simulink model "energy_recovery_testbench_r2024a"  (R2024a)
settings: Solver=daessc  StartTime=0  StopTime=0.4  MaxStep=1e-6  RelTol=1e-4
model workspace (MAT data in the model file):
  Fout_Hz = 50
  LoadEnable = 0
  RegenCurrentRef_RMS_A = 0.5
  RegenEnable = 1
  Rphase = 9.23760430703
libraries: fl_lib x38, nesl_utility x28
settings Model: Creator=chidan  LastModifiedBy=chidan

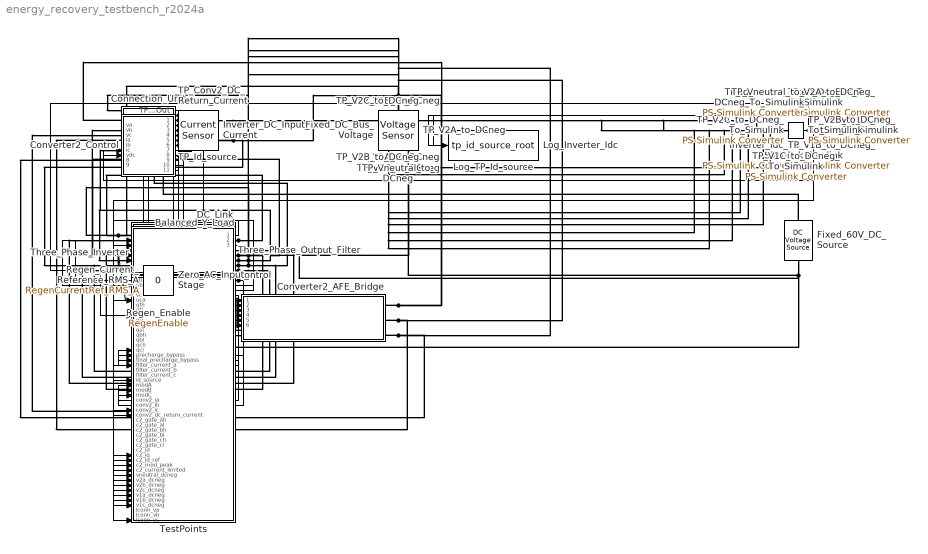
== system energy_recovery_testbench_r2024a ==
  Balanced_Y_Load : Subsystem
  Connection_Unit : Subsystem
  Control : Subsystem  ReferencedSubsystem=converter1_control_r2024a
  Converter2_AFE_Bridge : Subsystem  ReferencedSubsystem=converter1_inverter_r2024a
  Converter2_Control : Subsystem
  DC_Link : Subsystem
  Fixed_60V_DC_Source : fl_lib/Electrical/Electrical Sources/DC Voltage Source  v0=60 V
  Fixed_DC_Bus_To_Simulink : nesl_utility/PS-Simulink Converter  PhysicalDomain=network_engine_domain  SubClassName=ps_output  LeftPortType=input  RightPortType=output  PseudoPeriodic=off  Frequencies=[]  VectorFormat=inherit  Unit=V  AffineConversion=off
  Fixed_DC_Bus_Voltage : fl_lib/Electrical/Electrical Sensors/Voltage Sensor
  Inverter_DC_Input_Current : fl_lib/Electrical/Electrical Sensors/Current Sensor
  Inverter_Idc_To_Simulink : nesl_utility/PS-Simulink Converter  PhysicalDomain=network_engine_domain  SubClassName=ps_output  LeftPortType=input  RightPortType=output  PseudoPeriodic=off  Frequencies=[]  VectorFormat=inherit  Unit=A  AffineConversion=off
  Log_Inverter_Idc : ToWorkspace  VariableName=acac_idc_inverter  SaveFormat=Timeseries  SampleTime=-1
  Log_TP_Id_source : ToWorkspace  VariableName=tp_id_source_root  SaveFormat=Timeseries  SampleTime=-1
  Regen_Current_Reference_RMS_A : Constant  Value=RegenCurrentRef_RMS_A
  Regen_Enable : Constant  Value=RegenEnable
  TP_Conv2_DC_Return_Current : fl_lib/Electrical/Electrical Sensors/Current Sensor
  TP_Conv2_DC_Return_To_Simulink : nesl_utility/PS-Simulink Converter  PhysicalDomain=network_engine_domain  SubClassName=ps_output  LeftPortType=input  RightPortType=output  PseudoPeriodic=off  Frequencies=[]  VectorFormat=inherit  Unit=inherit  AffineConversion=off
  TP_Id_source : fl_lib/Electrical/Electrical Sensors/Current Sensor
  TP_Id_source_To_Simulink : nesl_utility/PS-Simulink Converter  PhysicalDomain=network_engine_domain  SubClassName=ps_output  LeftPortType=input  RightPortType=output  PseudoPeriodic=off  Frequencies=[]  VectorFormat=inherit  Unit=inherit  AffineConversion=off
  TP_V1A_to_DCneg : fl_lib/Electrical/Electrical Sensors/Voltage Sensor
  TP_V1A_to_DCneg_To_Simulink : nesl_utility/PS-Simulink Converter  PhysicalDomain=network_engine_domain  SubClassName=ps_output  LeftPortType=input  RightPortType=output  PseudoPeriodic=off  Frequencies=[]  VectorFormat=inherit  Unit=inherit  AffineConversion=off
  TP_V1B_to_DCneg : fl_lib/Electrical/Electrical Sensors/Voltage Sensor
  TP_V1B_to_DCneg_To_Simulink : nesl_utility/PS-Simulink Converter  PhysicalDomain=network_engine_domain  SubClassName=ps_output  LeftPortType=input  RightPortType=output  PseudoPeriodic=off  Frequencies=[]  VectorFormat=inherit  Unit=inherit  AffineConversion=off
  TP_V1C_to_DCneg : fl_lib/Electrical/Electrical Sensors/Voltage Sensor
  TP_V1C_to_DCneg_To_Simulink : nesl_utility/PS-Simulink Converter  PhysicalDomain=network_engine_domain  SubClassName=ps_output  LeftPortType=input  RightPortType=output  PseudoPeriodic=off  Frequencies=[]  VectorFormat=inherit  Unit=inherit  AffineConversion=off
  TP_V2A_to_DCneg : fl_lib/Electrical/Electrical Sensors/Voltage Sensor
  TP_V2A_to_DCneg_To_Simulink : nesl_utility/PS-Simulink Converter  PhysicalDomain=network_engine_domain  SubClassName=ps_output  LeftPortType=input  RightPortType=output  PseudoPeriodic=off  Frequencies=[]  VectorFormat=inherit  Unit=inherit  AffineConversion=off
  TP_V2B_to_DCneg : fl_lib/Electrical/Electrical Sensors/Voltage Sensor
  TP_V2B_to_DCneg_To_Simulink : nesl_utility/PS-Simulink Converter  PhysicalDomain=network_engine_domain  SubClassName=ps_output  LeftPortType=input  RightPortType=output  PseudoPeriodic=off  Frequencies=[]  VectorFormat=inherit  Unit=inherit  AffineConversion=off
  TP_V2C_to_DCneg : fl_lib/Electrical/Electrical Sensors/Voltage Sensor
  TP_V2C_to_DCneg_To_Simulink : nesl_utility/PS-Simulink Converter  PhysicalDomain=network_engine_domain  SubClassName=ps_output  LeftPortType=input  RightPortType=output  PseudoPeriodic=off  Frequencies=[]  VectorFormat=inherit  Unit=inherit  AffineConversion=off
  TP_Vneutral_to_DCneg : fl_lib/Electrical/Electrical Sensors/Voltage Sensor
  TP_Vneutral_to_DCneg_To_Simulink : nesl_utility/PS-Simulink Converter  PhysicalDomain=network_engine_domain  SubClassName=ps_output  LeftPortType=input  RightPortType=output  PseudoPeriodic=off  Frequencies=[]  VectorFormat=inherit  Unit=inherit  AffineConversion=off
  TestPoints : Subsystem
  Three_Phase_Inverter : Subsystem  ReferencedSubsystem=converter1_inverter_r2024a
  Three_Phase_Output_Filter : Subsystem  ReferencedSubsystem=converter1_filter_r2024a
  Zero_AC_Input_Stage : Constant  Value=0
  wires:
  Control/1 -> TestPoints/15(qfh)
  Control/2 -> TestPoints/16(qfl)
  Control/3 -> TestPoints/17(qsh)
  Control/4 -> TestPoints/18(qsl)
  Control/5 -> Three_Phase_Inverter/1, TestPoints/19(qah)
  Control/6 -> Three_Phase_Inverter/2, TestPoints/20(qal)
  Control/7 -> Three_Phase_Inverter/3, TestPoints/21(qbh)
  Control/8 -> Three_Phase_Inverter/4, TestPoints/22(qbl)
  Control/9 -> Three_Phase_Inverter/5, TestPoints/23(qch)
  Control/10 -> Three_Phase_Inverter/6, TestPoints/24(qcl)
  Balanced_Y_Load/2(Va) -> Control/4, TestPoints/7(va), Converter2_Control/1(va)
  Control/11 -> TestPoints/4(pfc_duty)
  Control/12 -> TestPoints/5(inverter_modulation)
  Balanced_Y_Load/1(Ia) -> TestPoints/6(ia)
  Balanced_Y_Load/3(Uab) -> TestPoints/8(uab)
  Balanced_Y_Load/4(Ib) -> TestPoints/9(ib)
  Balanced_Y_Load/5(Vb) -> TestPoints/10(vb), Control/5, Converter2_Control/2(vb)
  Balanced_Y_Load/6(Ubc) -> TestPoints/11(ubc)
  Balanced_Y_Load/7(Ic) -> TestPoints/12(ic)
  Balanced_Y_Load/8(Vc) -> TestPoints/13(vc), Control/6, Converter2_Control/3(vc)
  Balanced_Y_Load/9(Uca) -> TestPoints/14(uca)
  Control/13 -> TestPoints/25(precharge_bypass)
  Control/14 -> TestPoints/26(final_precharge_bypass)
  Inverter_Idc_To_Simulink/1 -> Log_Inverter_Idc/1
  Fixed_DC_Bus_To_Simulink/1 -> Control/3, TestPoints/3(vdc), Converter2_Control/7(vdc)
  Zero_AC_Input_Stage/1 -> Control/1, Control/2, TestPoints/1(vin), TestPoints/2(iin)
  TP_Id_source_To_Simulink/1 -> Log_TP_Id_source/1, TestPoints/30(id_source)
  Three_Phase_Output_Filter/1 -> TestPoints/27(filter_current_a)
  Three_Phase_Output_Filter/2 -> TestPoints/28(filter_current_b)
  Three_Phase_Output_Filter/3 -> TestPoints/29(filter_current_c)
  Control/15 -> TestPoints/31(modA)
  Control/16 -> TestPoints/32(modB)
  Control/17 -> TestPoints/33(modC)
  Connection_Unit/1(TP_Conv2_IA_Out) -> TestPoints/34(conv2_ia), Converter2_Control/4(ia)
  Connection_Unit/2(TP_Conv2_IB_Out) -> TestPoints/35(conv2_ib), Converter2_Control/5(ib)
  Connection_Unit/3(TP_Conv2_IC_Out) -> TestPoints/36(conv2_ic), Converter2_Control/6(ic)
  TP_Conv2_DC_Return_To_Simulink/1 -> TestPoints/37(conv2_dc_return_current)
  Regen_Current_Reference_RMS_A/1 -> Converter2_Control/8(iref_rms)
  Regen_Enable/1 -> Converter2_Control/9(regen_enable)
  Converter2_Control/1(Gate_AH) -> Converter2_AFE_Bridge/1, TestPoints/38(c2_gate_ah)
  Converter2_Control/2(Gate_AL) -> Converter2_AFE_Bridge/2, TestPoints/39(c2_gate_al)
  Converter2_Control/3(Gate_BH) -> Converter2_AFE_Bridge/3, TestPoints/40(c2_gate_bh)
  Converter2_Control/4(Gate_BL) -> Converter2_AFE_Bridge/4, TestPoints/41(c2_gate_bl)
  Converter2_Control/5(Gate_CH) -> Converter2_AFE_Bridge/5, TestPoints/42(c2_gate_ch)
  Converter2_Control/6(Gate_CL) -> Converter2_AFE_Bridge/6, TestPoints/43(c2_gate_cl)
  Converter2_Control/7(id_meas) -> TestPoints/44(c2_id)
  Converter2_Control/8(iq_meas) -> TestPoints/45(c2_iq)
  Converter2_Control/9(id_ref_used) -> TestPoints/46(c2_id_ref)
  Converter2_Control/10(mod_peak) -> TestPoints/47(c2_mod_peak)
  Converter2_Control/11(current_limited) -> TestPoints/48(c2_current_limited)
  TP_Vneutral_to_DCneg_To_Simulink/1 -> TestPoints/49(vneutral_dcneg)
  TP_V2A_to_DCneg_To_Simulink/1 -> TestPoints/50(v2a_dcneg)
  TP_V2B_to_DCneg_To_Simulink/1 -> TestPoints/51(v2b_dcneg)
  TP_V2C_to_DCneg_To_Simulink/1 -> TestPoints/52(v2c_dcneg)
  TP_V1A_to_DCneg_To_Simulink/1 -> TestPoints/53(v1a_dcneg)
  TP_V1B_to_DCneg_To_Simulink/1 -> TestPoints/54(v1b_dcneg)
  TP_V1C_to_DCneg_To_Simulink/1 -> TestPoints/55(v1c_dcneg)
  Connection_Unit/4(TP_Lconn_VA_Out) -> TestPoints/56(lconn_va)
  Connection_Unit/5(TP_Lconn_VB_Out) -> TestPoints/57(lconn_vb)
  Connection_Unit/6(TP_Lconn_VC_Out) -> TestPoints/58(lconn_vc)
  connections:
  Three_Phase_Inverter/RConn1 -- Three_Phase_Output_Filter/LConn1
  Three_Phase_Inverter/RConn2 -- Three_Phase_Output_Filter/LConn2
  Three_Phase_Inverter/RConn3 -- Three_Phase_Output_Filter/LConn3
  Balanced_Y_Load/LConn1 -- Three_Phase_Output_Filter/RConn1 -- Connection_Unit/LConn1 -- TP_V1A_to_DCneg/LConn1
  Balanced_Y_Load/LConn2 -- Three_Phase_Output_Filter/RConn2 -- Connection_Unit/LConn3 -- TP_V1B_to_DCneg/LConn1
  Balanced_Y_Load/LConn3 -- Three_Phase_Output_Filter/RConn3 -- Connection_Unit/LConn5 -- TP_V1C_to_DCneg/LConn1
  Balanced_Y_Load/LConn4 -- Three_Phase_Output_Filter/RConn4 -- TP_Vneutral_to_DCneg/LConn1
  Inverter_DC_Input_Current/RConn2 -- Three_Phase_Inverter/LConn1
  Inverter_DC_Input_Current/RConn1 -- Inverter_Idc_To_Simulink/LConn1
  Three_Phase_Inverter/LConn2 -- Fixed_60V_DC_Source/RConn1 -- Converter2_AFE_Bridge/LConn2 -- TP_Vneutral_to_DCneg/RConn2 -- TP_V2A_to_DCneg/RConn2 -- TP_V2B_to_DCneg/RConn2 -- TP_V2C_to_DCneg/RConn2 -- TP_V1A_to_DCneg/RConn2 -- TP_V1B_to_DCneg/RConn2 -- TP_V1C_to_DCneg/RConn2 -- DC_Link/LConn2 -- Fixed_DC_Bus_Voltage/RConn2
  Fixed_DC_Bus_Voltage/RConn1 -- Fixed_DC_Bus_To_Simulink/LConn1
  Fixed_60V_DC_Source/LConn1 -- TP_Id_source/LConn1
  TP_Id_source/RConn1 -- TP_Id_source_To_Simulink/LConn1
  Converter2_AFE_Bridge/RConn1 -- Connection_Unit/LConn2 -- TP_V2A_to_DCneg/LConn1
  Converter2_AFE_Bridge/RConn2 -- Connection_Unit/LConn4 -- TP_V2B_to_DCneg/LConn1
  Converter2_AFE_Bridge/RConn3 -- Connection_Unit/LConn6 -- TP_V2C_to_DCneg/LConn1
  DC_Link/LConn1 -- Inverter_DC_Input_Current/LConn1 -- Fixed_DC_Bus_Voltage/LConn1 -- TP_Conv2_DC_Return_Current/RConn2 -- TP_Id_source/RConn2
  Converter2_AFE_Bridge/LConn1 -- TP_Conv2_DC_Return_Current/LConn1
  TP_Conv2_DC_Return_Current/RConn1 -- TP_Conv2_DC_Return_To_Simulink/LConn1
  TP_Vneutral_to_DCneg/RConn1 -- TP_Vneutral_to_DCneg_To_Simulink/LConn1
  TP_V2A_to_DCneg/RConn1 -- TP_V2A_to_DCneg_To_Simulink/LConn1
  TP_V2B_to_DCneg/RConn1 -- TP_V2B_to_DCneg_To_Simulink/LConn1
  TP_V2C_to_DCneg/RConn1 -- TP_V2C_to_DCneg_To_Simulink/LConn1
  TP_V1A_to_DCneg/RConn1 -- TP_V1A_to_DCneg_To_Simulink/LConn1
  TP_V1B_to_DCneg/RConn1 -- TP_V1B_to_DCneg_To_Simulink/LConn1
  TP_V1C_to_DCneg/RConn1 -- TP_V1C_to_DCneg_To_Simulink/LConn1

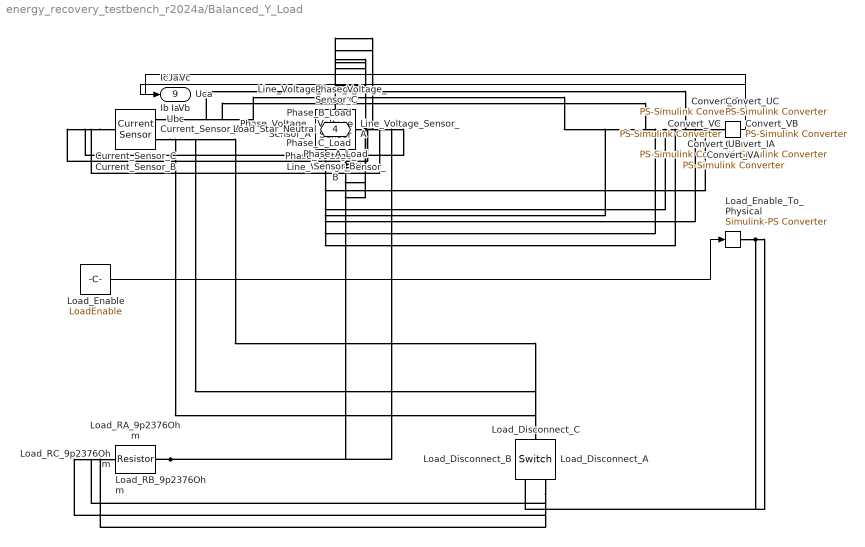
== system energy_recovery_testbench_r2024a/Balanced_Y_Load ==
  Convert_IA : nesl_utility/PS-Simulink Converter  PhysicalDomain=network_engine_domain  SubClassName=ps_output  LeftPortType=input  RightPortType=output  PseudoPeriodic=off  Frequencies=[]  VectorFormat=inherit  Unit=inherit  AffineConversion=off
  Convert_IB : nesl_utility/PS-Simulink Converter  PhysicalDomain=network_engine_domain  SubClassName=ps_output  LeftPortType=input  RightPortType=output  PseudoPeriodic=off  Frequencies=[]  VectorFormat=inherit  Unit=inherit  AffineConversion=off
  Convert_IC : nesl_utility/PS-Simulink Converter  PhysicalDomain=network_engine_domain  SubClassName=ps_output  LeftPortType=input  RightPortType=output  PseudoPeriodic=off  Frequencies=[]  VectorFormat=inherit  Unit=inherit  AffineConversion=off
  Convert_UA : nesl_utility/PS-Simulink Converter  PhysicalDomain=network_engine_domain  SubClassName=ps_output  LeftPortType=input  RightPortType=output  PseudoPeriodic=off  Frequencies=[]  VectorFormat=inherit  Unit=inherit  AffineConversion=off
  Convert_UB : nesl_utility/PS-Simulink Converter  PhysicalDomain=network_engine_domain  SubClassName=ps_output  LeftPortType=input  RightPortType=output  PseudoPeriodic=off  Frequencies=[]  VectorFormat=inherit  Unit=inherit  AffineConversion=off
  Convert_UC : nesl_utility/PS-Simulink Converter  PhysicalDomain=network_engine_domain  SubClassName=ps_output  LeftPortType=input  RightPortType=output  PseudoPeriodic=off  Frequencies=[]  VectorFormat=inherit  Unit=inherit  AffineConversion=off
  Convert_VA : nesl_utility/PS-Simulink Converter  PhysicalDomain=network_engine_domain  SubClassName=ps_output  LeftPortType=input  RightPortType=output  PseudoPeriodic=off  Frequencies=[]  VectorFormat=inherit  Unit=inherit  AffineConversion=off
  Convert_VB : nesl_utility/PS-Simulink Converter  PhysicalDomain=network_engine_domain  SubClassName=ps_output  LeftPortType=input  RightPortType=output  PseudoPeriodic=off  Frequencies=[]  VectorFormat=inherit  Unit=inherit  AffineConversion=off
  Convert_VC : nesl_utility/PS-Simulink Converter  PhysicalDomain=network_engine_domain  SubClassName=ps_output  LeftPortType=input  RightPortType=output  PseudoPeriodic=off  Frequencies=[]  VectorFormat=inherit  Unit=inherit  AffineConversion=off
  Current_Sensor_A : fl_lib/Electrical/Electrical Sensors/Current Sensor
  Current_Sensor_B : fl_lib/Electrical/Electrical Sensors/Current Sensor
  Current_Sensor_C : fl_lib/Electrical/Electrical Sensors/Current Sensor
  Line_Voltage_Sensor_A : fl_lib/Electrical/Electrical Sensors/Voltage Sensor
  Line_Voltage_Sensor_B : fl_lib/Electrical/Electrical Sensors/Voltage Sensor
  Line_Voltage_Sensor_C : fl_lib/Electrical/Electrical Sensors/Voltage Sensor
  Load_Disconnect_A : fl_lib/Electrical/Electrical Elements/Switch  R_closed=0.001 Ohm  G_open=1e-12 1/Ohm  Threshold=0.5  i_specify=off  i_priority=None  i=0 A  i_nominal_specify=off  i_nominal_value=1  i_nominal_unit=A  v_specify=off  v_priority=None  v=0 V  v_nominal_specify=off  v_nominal_value=1  v_nominal_unit=V
  Load_Disconnect_B : fl_lib/Electrical/Electrical Elements/Switch  R_closed=0.001 Ohm  G_open=1e-12 1/Ohm  Threshold=0.5  i_specify=off  i_priority=None  i=0 A  i_nominal_specify=off  i_nominal_value=1  i_nominal_unit=A  v_specify=off  v_priority=None  v=0 V  v_nominal_specify=off  v_nominal_value=1  v_nominal_unit=V
  Load_Disconnect_C : fl_lib/Electrical/Electrical Elements/Switch  R_closed=0.001 Ohm  G_open=1e-12 1/Ohm  Threshold=0.5  i_specify=off  i_priority=None  i=0 A  i_nominal_specify=off  i_nominal_value=1  i_nominal_unit=A  v_specify=off  v_priority=None  v=0 V  v_nominal_specify=off  v_nominal_value=1  v_nominal_unit=V
  Load_Enable : Constant  Value=LoadEnable
  Load_Enable_To_Physical : nesl_utility/Simulink-PS Converter  PhysicalDomain=network_engine_domain  SubClassName=ps_input  LeftPortType=input  RightPortType=output  PseudoPeriodic=off  Frequencies=[]  NoiseDistribution=none  NoiseParameters=[]  Unit=1  AffineConversion=off  FilteringAndDerivatives=provide  SimscapeFilterOrder=1  InputFilterTimeConstant=0.001  UdotUserProvided=0
  Load_RA_9p2376Ohm : fl_lib/Electrical/Electrical Elements/Resistor  R=Rphase Ohm  i_specify=off  i_priority=None  i=0 A  i_nominal_specify=off  i_nominal_value=1  i_nominal_unit=A  v_specify=off  v_priority=None  v=0 V  v_nominal_specify=off  v_nominal_value=1  v_nominal_unit=V
  Load_RB_9p2376Ohm : fl_lib/Electrical/Electrical Elements/Resistor  R=Rphase Ohm  i_specify=off  i_priority=None  i=0 A  i_nominal_specify=off  i_nominal_value=1  i_nominal_unit=A  v_specify=off  v_priority=None  v=0 V  v_nominal_specify=off  v_nominal_value=1  v_nominal_unit=V
  Load_RC_9p2376Ohm : fl_lib/Electrical/Electrical Elements/Resistor  R=Rphase Ohm  i_specify=off  i_priority=None  i=0 A  i_nominal_specify=off  i_nominal_value=1  i_nominal_unit=A  v_specify=off  v_priority=None  v=0 V  v_nominal_specify=off  v_nominal_value=1  v_nominal_unit=V
  Phase_Voltage_Sensor_A : fl_lib/Electrical/Electrical Sensors/Voltage Sensor
  Phase_Voltage_Sensor_B : fl_lib/Electrical/Electrical Sensors/Voltage Sensor
  Phase_Voltage_Sensor_C : fl_lib/Electrical/Electrical Sensors/Voltage Sensor
  Phase_A_Load : PMIOPort  Side=Left
  Phase_B_Load : PMIOPort  Port=2  Side=Left
  Phase_C_Load : PMIOPort  Port=3  Side=Left
  Load_Star_Neutral : PMIOPort  Port=4  Side=Left
  Ia : Outport
  Va : Outport  Port=2
  Uab : Outport  Port=3
  Ib : Outport  Port=4
  Vb : Outport  Port=5
  Ubc : Outport  Port=6
  Ic : Outport  Port=7
  Vc : Outport  Port=8
  Uca : Outport  Port=9
  wires:
  Convert_IA/1 -> Ia/1
  Convert_VA/1 -> Va/1
  Convert_IB/1 -> Ib/1
  Convert_VB/1 -> Vb/1
  Convert_IC/1 -> Ic/1
  Convert_VC/1 -> Vc/1
  Convert_UA/1 -> Uab/1
  Convert_UB/1 -> Ubc/1
  Convert_UC/1 -> Uca/1
  Load_Enable/1 -> Load_Enable_To_Physical/1
  connections:
  Current_Sensor_A/LConn1 -- Phase_A_Load/RConn1 -- Phase_Voltage_Sensor_A/LConn1 -- Line_Voltage_Sensor_A/LConn1 -- Line_Voltage_Sensor_C/RConn2
  Phase_Voltage_Sensor_A/RConn2 -- Load_Star_Neutral/RConn1 -- Load_RA_9p2376Ohm/RConn1 -- Phase_Voltage_Sensor_B/RConn2 -- Phase_Voltage_Sensor_C/RConn2 -- Load_RB_9p2376Ohm/RConn1 -- Load_RC_9p2376Ohm/RConn1
  Current_Sensor_B/LConn1 -- Phase_B_Load/RConn1 -- Phase_Voltage_Sensor_B/LConn1 -- Line_Voltage_Sensor_A/RConn2 -- Line_Voltage_Sensor_B/LConn1
  Current_Sensor_C/LConn1 -- Phase_C_Load/RConn1 -- Phase_Voltage_Sensor_C/LConn1 -- Line_Voltage_Sensor_B/RConn2 -- Line_Voltage_Sensor_C/LConn1
  Current_Sensor_A/RConn1 -- Convert_IA/LConn1
  Current_Sensor_B/RConn1 -- Convert_IB/LConn1
  Current_Sensor_C/RConn1 -- Convert_IC/LConn1
  Phase_Voltage_Sensor_A/RConn1 -- Convert_VA/LConn1
  Phase_Voltage_Sensor_B/RConn1 -- Convert_VB/LConn1
  Phase_Voltage_Sensor_C/RConn1 -- Convert_VC/LConn1
  Line_Voltage_Sensor_A/RConn1 -- Convert_UA/LConn1
  Line_Voltage_Sensor_B/RConn1 -- Convert_UB/LConn1
  Line_Voltage_Sensor_C/RConn1 -- Convert_UC/LConn1
  Current_Sensor_A/RConn2 -- Load_Disconnect_A/LConn1
  Load_Disconnect_A/RConn2 -- Load_RA_9p2376Ohm/LConn1
  Current_Sensor_B/RConn2 -- Load_Disconnect_B/LConn1
  Load_Disconnect_B/RConn2 -- Load_RB_9p2376Ohm/LConn1
  Current_Sensor_C/RConn2 -- Load_Disconnect_C/LConn1
  Load_Disconnect_C/RConn2 -- Load_RC_9p2376Ohm/LConn1
  Load_Disconnect_A/RConn1 -- Load_Enable_To_Physical/RConn1 -- Load_Disconnect_B/RConn1 -- Load_Disconnect_C/RConn1

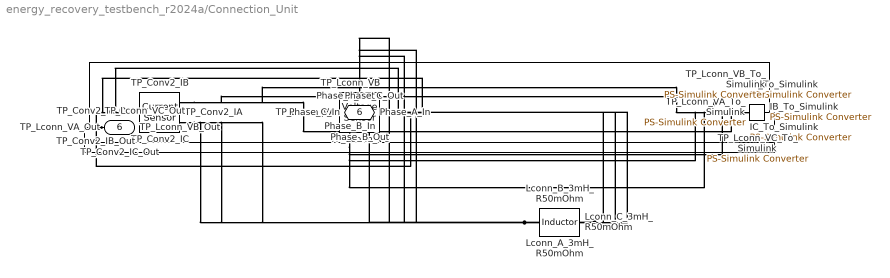
== system energy_recovery_testbench_r2024a/Connection_Unit ==
  IA_To_Simulink : nesl_utility/PS-Simulink Converter  PhysicalDomain=network_engine_domain  SubClassName=ps_output  LeftPortType=input  RightPortType=output  PseudoPeriodic=off  Frequencies=[]  VectorFormat=inherit  Unit=inherit  AffineConversion=off
  IB_To_Simulink : nesl_utility/PS-Simulink Converter  PhysicalDomain=network_engine_domain  SubClassName=ps_output  LeftPortType=input  RightPortType=output  PseudoPeriodic=off  Frequencies=[]  VectorFormat=inherit  Unit=inherit  AffineConversion=off
  IC_To_Simulink : nesl_utility/PS-Simulink Converter  PhysicalDomain=network_engine_domain  SubClassName=ps_output  LeftPortType=input  RightPortType=output  PseudoPeriodic=off  Frequencies=[]  VectorFormat=inherit  Unit=inherit  AffineConversion=off
  Lconn_A_3mH_R50mOhm : fl_lib/Electrical/Electrical Elements/Inductor  l=0.003 H  r=0.05 Ohm  g=1e-9 1/Ohm  i_specify=off  i_priority=None  i=0 A  i_nominal_specify=off  i_nominal_value=1  i_nominal_unit=A  v_specify=off  v_priority=None  v=0 V  v_nominal_specify=off  v_nominal_value=1  v_nominal_unit=V  i_L_specify=off  i_L_priority=High  i_L=0 A  i_L_nominal_specify=off  i_L_nominal_value=1  i_L_nominal_unit=A
  Lconn_B_3mH_R50mOhm : fl_lib/Electrical/Electrical Elements/Inductor  l=0.003 H  r=0.05 Ohm  g=1e-9 1/Ohm  i_specify=off  i_priority=None  i=0 A  i_nominal_specify=off  i_nominal_value=1  i_nominal_unit=A  v_specify=off  v_priority=None  v=0 V  v_nominal_specify=off  v_nominal_value=1  v_nominal_unit=V  i_L_specify=off  i_L_priority=High  i_L=0 A  i_L_nominal_specify=off  i_L_nominal_value=1  i_L_nominal_unit=A
  Lconn_C_3mH_R50mOhm : fl_lib/Electrical/Electrical Elements/Inductor  l=0.003 H  r=0.05 Ohm  g=1e-9 1/Ohm  i_specify=off  i_priority=None  i=0 A  i_nominal_specify=off  i_nominal_value=1  i_nominal_unit=A  v_specify=off  v_priority=None  v=0 V  v_nominal_specify=off  v_nominal_value=1  v_nominal_unit=V  i_L_specify=off  i_L_priority=High  i_L=0 A  i_L_nominal_specify=off  i_L_nominal_value=1  i_L_nominal_unit=A
  TP_Conv2_IA : fl_lib/Electrical/Electrical Sensors/Current Sensor
  TP_Conv2_IB : fl_lib/Electrical/Electrical Sensors/Current Sensor
  TP_Conv2_IC : fl_lib/Electrical/Electrical Sensors/Current Sensor
  TP_Lconn_VA : fl_lib/Electrical/Electrical Sensors/Voltage Sensor
  TP_Lconn_VA_To_Simulink : nesl_utility/PS-Simulink Converter  PhysicalDomain=network_engine_domain  SubClassName=ps_output  LeftPortType=input  RightPortType=output  PseudoPeriodic=off  Frequencies=[]  VectorFormat=inherit  Unit=inherit  AffineConversion=off
  TP_Lconn_VB : fl_lib/Electrical/Electrical Sensors/Voltage Sensor
  TP_Lconn_VB_To_Simulink : nesl_utility/PS-Simulink Converter  PhysicalDomain=network_engine_domain  SubClassName=ps_output  LeftPortType=input  RightPortType=output  PseudoPeriodic=off  Frequencies=[]  VectorFormat=inherit  Unit=inherit  AffineConversion=off
  TP_Lconn_VC : fl_lib/Electrical/Electrical Sensors/Voltage Sensor
  TP_Lconn_VC_To_Simulink : nesl_utility/PS-Simulink Converter  PhysicalDomain=network_engine_domain  SubClassName=ps_output  LeftPortType=input  RightPortType=output  PseudoPeriodic=off  Frequencies=[]  VectorFormat=inherit  Unit=inherit  AffineConversion=off
  Phase_A_In : PMIOPort  Side=Left
  Phase_A_Out : PMIOPort  Port=2  Side=Left
  Phase_B_In : PMIOPort  Port=3  Side=Left
  Phase_B_Out : PMIOPort  Port=4  Side=Left
  Phase_C_In : PMIOPort  Port=5  Side=Left
  Phase_C_Out : PMIOPort  Port=6  Side=Left
  TP_Conv2_IA_Out : Outport
  TP_Conv2_IB_Out : Outport  Port=2
  TP_Conv2_IC_Out : Outport  Port=3
  TP_Lconn_VA_Out : Outport  Port=4
  TP_Lconn_VB_Out : Outport  Port=5
  TP_Lconn_VC_Out : Outport  Port=6
  wires:
  IA_To_Simulink/1 -> TP_Conv2_IA_Out/1
  IB_To_Simulink/1 -> TP_Conv2_IB_Out/1
  IC_To_Simulink/1 -> TP_Conv2_IC_Out/1
  TP_Lconn_VA_To_Simulink/1 -> TP_Lconn_VA_Out/1
  TP_Lconn_VB_To_Simulink/1 -> TP_Lconn_VB_Out/1
  TP_Lconn_VC_To_Simulink/1 -> TP_Lconn_VC_Out/1
  connections:
  Phase_A_In/RConn1 -- TP_Conv2_IA/LConn1
  Lconn_A_3mH_R50mOhm/LConn1 -- TP_Conv2_IA/RConn2 -- TP_Lconn_VA/LConn1
  Phase_A_Out/RConn1 -- Lconn_A_3mH_R50mOhm/RConn1 -- TP_Lconn_VA/RConn2
  TP_Conv2_IA/RConn1 -- IA_To_Simulink/LConn1
  Phase_B_In/RConn1 -- TP_Conv2_IB/LConn1
  Lconn_B_3mH_R50mOhm/LConn1 -- TP_Conv2_IB/RConn2 -- TP_Lconn_VB/LConn1
  Phase_B_Out/RConn1 -- Lconn_B_3mH_R50mOhm/RConn1 -- TP_Lconn_VB/RConn2
  TP_Conv2_IB/RConn1 -- IB_To_Simulink/LConn1
  Phase_C_In/RConn1 -- TP_Conv2_IC/LConn1
  Lconn_C_3mH_R50mOhm/LConn1 -- TP_Conv2_IC/RConn2 -- TP_Lconn_VC/LConn1
  Phase_C_Out/RConn1 -- Lconn_C_3mH_R50mOhm/RConn1 -- TP_Lconn_VC/RConn2
  TP_Conv2_IC/RConn1 -- IC_To_Simulink/LConn1
  TP_Lconn_VA/RConn1 -- TP_Lconn_VA_To_Simulink/LConn1
  TP_Lconn_VB/RConn1 -- TP_Lconn_VB_To_Simulink/LConn1
  TP_Lconn_VC/RConn1 -- TP_Lconn_VC_To_Simulink/LConn1

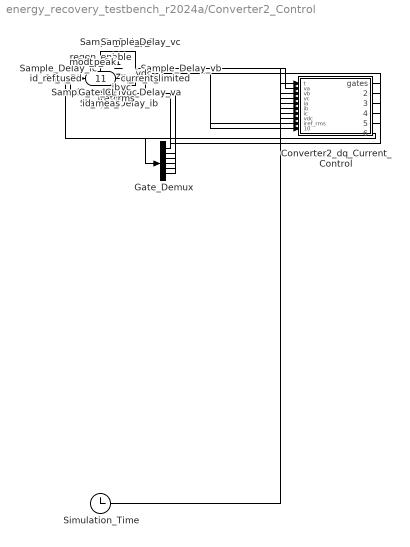
== system energy_recovery_testbench_r2024a/Converter2_Control ==
  va : Inport
  vb : Inport  Port=2
  vc : Inport  Port=3
  ia : Inport  Port=4
  ib : Inport  Port=5
  ic : Inport  Port=6
  vdc : Inport  Port=7
  iref_rms : Inport  Port=8
  regen_enable : Inport  Port=9
  Converter2_dq_Current_Control : MATLAB Function  TreatAsAtomicUnit=on
  Gate_Demux : Demux  Outputs=6
  Sample_Delay_ia : UnitDelay  SampleTime=1e-6  HasFrameUpgradeWarning=on
  Sample_Delay_ib : UnitDelay  SampleTime=1e-6  HasFrameUpgradeWarning=on
  Sample_Delay_ic : UnitDelay  SampleTime=1e-6  HasFrameUpgradeWarning=on
  Sample_Delay_va : UnitDelay  SampleTime=1e-6  HasFrameUpgradeWarning=on
  Sample_Delay_vb : UnitDelay  SampleTime=1e-6  HasFrameUpgradeWarning=on
  Sample_Delay_vc : UnitDelay  SampleTime=1e-6  HasFrameUpgradeWarning=on
  Sample_Delay_vdc : UnitDelay  SampleTime=1e-6  HasFrameUpgradeWarning=on
  Simulation_Time : Clock
  Gate_AH : Outport
  Gate_AL : Outport  Port=2
  Gate_BH : Outport  Port=3
  Gate_BL : Outport  Port=4
  Gate_CH : Outport  Port=5
  Gate_CL : Outport  Port=6
  id_meas : Outport  Port=7
  iq_meas : Outport  Port=8
  id_ref_used : Outport  Port=9
  mod_peak : Outport  Port=10
  current_limited : Outport  Port=11
  wires:
  va/1 -> Sample_Delay_va/1
  Sample_Delay_va/1 -> Converter2_dq_Current_Control/2(va)
  vb/1 -> Sample_Delay_vb/1
  Sample_Delay_vb/1 -> Converter2_dq_Current_Control/3(vb)
  vc/1 -> Sample_Delay_vc/1
  Sample_Delay_vc/1 -> Converter2_dq_Current_Control/4(vc)
  ia/1 -> Sample_Delay_ia/1
  Sample_Delay_ia/1 -> Converter2_dq_Current_Control/5(ia)
  ib/1 -> Sample_Delay_ib/1
  Sample_Delay_ib/1 -> Converter2_dq_Current_Control/6(ib)
  ic/1 -> Sample_Delay_ic/1
  Sample_Delay_ic/1 -> Converter2_dq_Current_Control/7(ic)
  vdc/1 -> Sample_Delay_vdc/1
  Sample_Delay_vdc/1 -> Converter2_dq_Current_Control/8(vdc)
  Simulation_Time/1 -> Converter2_dq_Current_Control/1(t)
  iref_rms/1 -> Converter2_dq_Current_Control/9(iref_rms)
  regen_enable/1 -> Converter2_dq_Current_Control/10(regen_enable)
  Converter2_dq_Current_Control/1(gates) -> Gate_Demux/1
  Gate_Demux/1 -> Gate_AH/1
  Gate_Demux/2 -> Gate_AL/1
  Gate_Demux/3 -> Gate_BH/1
  Gate_Demux/4 -> Gate_BL/1
  Gate_Demux/5 -> Gate_CH/1
  Gate_Demux/6 -> Gate_CL/1
  Converter2_dq_Current_Control/2(id_meas) -> id_meas/1
  Converter2_dq_Current_Control/3(iq_meas) -> iq_meas/1
  Converter2_dq_Current_Control/4(id_ref_used) -> id_ref_used/1
  Converter2_dq_Current_Control/5(mod_peak) -> mod_peak/1
  Converter2_dq_Current_Control/6(current_limited) -> current_limited/1

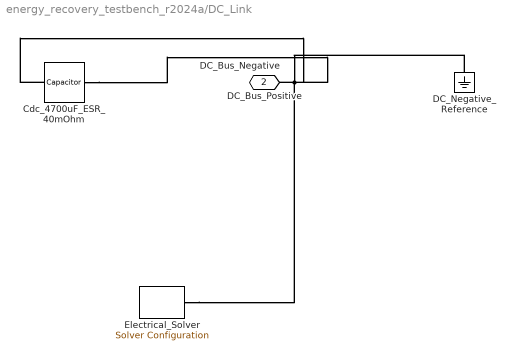
== system energy_recovery_testbench_r2024a/DC_Link ==
  Cdc_4700uF_ESR_40mOhm : fl_lib/Electrical/Electrical Elements/Capacitor  c=4.7e-3 F  r=0.04 Ohm  g=0 1/Ohm  i_specify=off  i_priority=None  i=0 A  i_nominal_specify=off  i_nominal_value=1  i_nominal_unit=A  v_specify=off  v_priority=None  v=0 V  v_nominal_specify=off  v_nominal_value=1  v_nominal_unit=V  vc_specify=off  vc_priority=High  vc=0 V  vc_nominal_specify=off  vc_nominal_value=1  vc_nominal_unit=V
  DC_Negative_Reference : fl_lib/Electrical/Electrical Elements/Electrical Reference
  Electrical_Solver : nesl_utility/Solver Configuration  PhysicalDomain=network_engine_domain  SubClassName=solver  LeftPortType=input  RightPortType=generic  Tones=[]  Harmonics=[]  SimulateNoise=off  Profile=off  UseLocalSampling=off  EnableSwitchedLinearOptims=on  FrequencyDomain=off  UseCCode=off  RelTol=0.001  AbsTol=0.001  MinStep=1e-09  ToWorkspace=off  RevertToSquareIcSolve=off  NumHomotopyIterations=100  PhasorMode=off  PhasorModeNumHarmonics=1  ConsistencySolver=NEWTON_XTOL_AFTER_FTOL  IndexReductionMethod=DerivativeReplacement  DoDC=off  ResidualTolerance=1e-09  ConsistencyTolSource=GLOBAL  ConsistencyAbsTol=0.001  ConsistencyRelTol=0.001  ConsistencyTolFactor=0.001  UseLocalSolver=off  LocalSolverChoice=NE_BACKWARD_EULER_ADVANCER  ResolveIndetEquations=on  FunctionEvalNumThread=1  LocalSolverSampleTime=0.001  DoFixedCost=off  MaxNonlinIter=3  MaxModeIter=2  ComputeImpulses=off  ImpulseIterations=2  LinearAlgebra=auto  LinearAlgebraNumThread=0  EquationFormulation=NE_TIME_EF  DelaysMemoryBudget=1024  AutomaticFiltering=on  FilteringTimeConstant=0.001  PartitionStorageMethod=AS_NEEDED  PartitionMemoryBudget=1024  PartitionMethod=ROBUST  MultibodyUseLocalSolver=off  MultibodyLocalSolverChoice=ODE1  MultibodyLocalSolverSampleTime=0.001
  DC_Bus_Positive : PMIOPort  Side=Left
  DC_Bus_Negative : PMIOPort  Port=2  Side=Left
  connections:
  Cdc_4700uF_ESR_40mOhm/LConn1 -- DC_Bus_Positive/RConn1
  Cdc_4700uF_ESR_40mOhm/RConn1 -- DC_Negative_Reference/LConn1 -- DC_Bus_Negative/RConn1 -- Electrical_Solver/RConn1

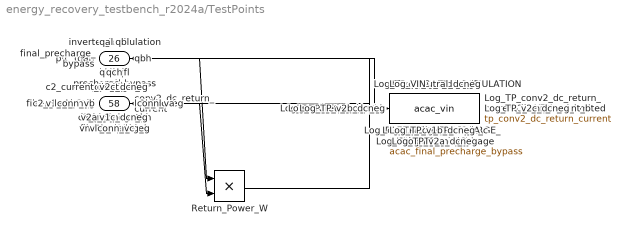
== system energy_recovery_testbench_r2024a/TestPoints ==
  vin : Inport
  iin : Inport  Port=2
  vdc : Inport  Port=3
  pfc_duty : Inport  Port=4
  inverter_modulation : Inport  Port=5
  ia : Inport  Port=6
  va : Inport  Port=7
  uab : Inport  Port=8
  ib : Inport  Port=9
  vb : Inport  Port=10
  ubc : Inport  Port=11
  ic : Inport  Port=12
  vc : Inport  Port=13
  uca : Inport  Port=14
  qfh : Inport  Port=15
  qfl : Inport  Port=16
  qsh : Inport  Port=17
  qsl : Inport  Port=18
  qah : Inport  Port=19
  qal : Inport  Port=20
  qbh : Inport  Port=21
  qbl : Inport  Port=22
  qch : Inport  Port=23
  qcl : Inport  Port=24
  precharge_bypass : Inport  Port=25
  final_precharge_bypass : Inport  Port=26
  filter_current_a : Inport  Port=27
  filter_current_b : Inport  Port=28
  filter_current_c : Inport  Port=29
  id_source : Inport  Port=30
  modA : Inport  Port=31
  modB : Inport  Port=32
  modC : Inport  Port=33
  conv2_ia : Inport  Port=34
  conv2_ib : Inport  Port=35
  conv2_ic : Inport  Port=36
  conv2_dc_return_current : Inport  Port=37
  c2_gate_ah : Inport  Port=38
  c2_gate_al : Inport  Port=39
  c2_gate_bh : Inport  Port=40
  c2_gate_bl : Inport  Port=41
  c2_gate_ch : Inport  Port=42
  c2_gate_cl : Inport  Port=43
  c2_id : Inport  Port=44
  c2_iq : Inport  Port=45
  c2_id_ref : Inport  Port=46
  c2_mod_peak : Inport  Port=47
  c2_current_limited : Inport  Port=48
  vneutral_dcneg : Inport  Port=49
  v2a_dcneg : Inport  Port=50
  v2b_dcneg : Inport  Port=51
  v2c_dcneg : Inport  Port=52
  v1a_dcneg : Inport  Port=53
  v1b_dcneg : Inport  Port=54
  v1c_dcneg : Inport  Port=55
  lconn_va : Inport  Port=56
  lconn_vb : Inport  Port=57
  lconn_vc : Inport  Port=58
  Log_FINAL_PRECHARGE_BYPASS : ToWorkspace  VariableName=acac_final_precharge_bypass  SaveFormat=Timeseries  SampleTime=-1
  Log_IA : ToWorkspace  VariableName=acac_ia  SaveFormat=Timeseries  SampleTime=-1
  Log_IB : ToWorkspace  VariableName=acac_ib  SaveFormat=Timeseries  SampleTime=-1
  Log_IC : ToWorkspace  VariableName=acac_ic  SaveFormat=Timeseries  SampleTime=-1
  Log_IIN : ToWorkspace  VariableName=acac_iin  SaveFormat=Timeseries  SampleTime=-1
  Log_INVERTER_MODULATION : ToWorkspace  VariableName=acac_inverter_modulation  SaveFormat=Timeseries  SampleTime=-1
  Log_PFC_DUTY : ToWorkspace  VariableName=acac_pfc_duty  SaveFormat=Timeseries  SampleTime=-1
  Log_PRECHARGE_BYPASS : ToWorkspace  VariableName=acac_precharge_bypass  SaveFormat=Timeseries  SampleTime=-1
  Log_QAH : ToWorkspace  VariableName=acac_qah  SaveFormat=Timeseries  SampleTime=-1
  Log_QAL : ToWorkspace  VariableName=acac_qal  SaveFormat=Timeseries  SampleTime=-1
  Log_QBH : ToWorkspace  VariableName=acac_qbh  SaveFormat=Timeseries  SampleTime=-1
  Log_QBL : ToWorkspace  VariableName=acac_qbl  SaveFormat=Timeseries  SampleTime=-1
  Log_QCH : ToWorkspace  VariableName=acac_qch  SaveFormat=Timeseries  SampleTime=-1
  Log_QCL : ToWorkspace  VariableName=acac_qcl  SaveFormat=Timeseries  SampleTime=-1
  Log_QFH : ToWorkspace  VariableName=acac_qfh  SaveFormat=Timeseries  SampleTime=-1
  Log_QFL : ToWorkspace  VariableName=acac_qfl  SaveFormat=Timeseries  SampleTime=-1
  Log_QSH : ToWorkspace  VariableName=acac_qsh  SaveFormat=Timeseries  SampleTime=-1
  Log_QSL : ToWorkspace  VariableName=acac_qsl  SaveFormat=Timeseries  SampleTime=-1
  Log_TP_c2_current_limited : ToWorkspace  VariableName=tp_c2_current_limited  SaveFormat=Timeseries  SampleTime=-1
  Log_TP_c2_gate_ah : ToWorkspace  VariableName=tp_c2_gate_ah  SaveFormat=Timeseries  SampleTime=-1
  Log_TP_c2_gate_al : ToWorkspace  VariableName=tp_c2_gate_al  SaveFormat=Timeseries  SampleTime=-1
  Log_TP_c2_gate_bh : ToWorkspace  VariableName=tp_c2_gate_bh  SaveFormat=Timeseries  SampleTime=-1
  Log_TP_c2_gate_bl : ToWorkspace  VariableName=tp_c2_gate_bl  SaveFormat=Timeseries  SampleTime=-1
  Log_TP_c2_gate_ch : ToWorkspace  VariableName=tp_c2_gate_ch  SaveFormat=Timeseries  SampleTime=-1
  Log_TP_c2_gate_cl : ToWorkspace  VariableName=tp_c2_gate_cl  SaveFormat=Timeseries  SampleTime=-1
  Log_TP_c2_id : ToWorkspace  VariableName=tp_c2_id  SaveFormat=Timeseries  SampleTime=-1
  Log_TP_c2_id_ref : ToWorkspace  VariableName=tp_c2_id_ref  SaveFormat=Timeseries  SampleTime=-1
  Log_TP_c2_iq : ToWorkspace  VariableName=tp_c2_iq  SaveFormat=Timeseries  SampleTime=-1
  Log_TP_c2_mod_peak : ToWorkspace  VariableName=tp_c2_mod_peak  SaveFormat=Timeseries  SampleTime=-1
  Log_TP_conv2_dc_return_current : ToWorkspace  VariableName=tp_conv2_dc_return_current  SaveFormat=Timeseries  SampleTime=-1
  Log_TP_conv2_dc_voltage : ToWorkspace  VariableName=tp_conv2_dc_voltage  SaveFormat=Timeseries  SampleTime=-1
  Log_TP_conv2_ia : ToWorkspace  VariableName=tp_conv2_ia  SaveFormat=Timeseries  SampleTime=-1
  Log_TP_conv2_ib : ToWorkspace  VariableName=tp_conv2_ib  SaveFormat=Timeseries  SampleTime=-1
  Log_TP_conv2_ic : ToWorkspace  VariableName=tp_conv2_ic  SaveFormat=Timeseries  SampleTime=-1
  Log_TP_filter_current_a : ToWorkspace  VariableName=tp_filter_current_a  SaveFormat=Timeseries  SampleTime=-1
  Log_TP_filter_current_b : ToWorkspace  VariableName=tp_filter_current_b  SaveFormat=Timeseries  SampleTime=-1
  Log_TP_filter_current_c : ToWorkspace  VariableName=tp_filter_current_c  SaveFormat=Timeseries  SampleTime=-1
  Log_TP_id_source : ToWorkspace  VariableName=tp_id_source  SaveFormat=Timeseries  SampleTime=-1
  Log_TP_lconn_va : ToWorkspace  VariableName=tp_lconn_va  SaveFormat=Timeseries  SampleTime=-1
  Log_TP_lconn_vb : ToWorkspace  VariableName=tp_lconn_vb  SaveFormat=Timeseries  SampleTime=-1
  Log_TP_lconn_vc : ToWorkspace  VariableName=tp_lconn_vc  SaveFormat=Timeseries  SampleTime=-1
  Log_TP_modA : ToWorkspace  VariableName=tp_moda  SaveFormat=Timeseries  SampleTime=-1
  Log_TP_modB : ToWorkspace  VariableName=tp_modb  SaveFormat=Timeseries  SampleTime=-1
  Log_TP_modC : ToWorkspace  VariableName=tp_modc  SaveFormat=Timeseries  SampleTime=-1
  Log_TP_return_power : ToWorkspace  VariableName=tp_return_power  SaveFormat=Timeseries  SampleTime=-1
  Log_TP_v1a_dcneg : ToWorkspace  VariableName=tp_v1a_dcneg  SaveFormat=Timeseries  SampleTime=-1
  Log_TP_v1b_dcneg : ToWorkspace  VariableName=tp_v1b_dcneg  SaveFormat=Timeseries  SampleTime=-1
  Log_TP_v1c_dcneg : ToWorkspace  VariableName=tp_v1c_dcneg  SaveFormat=Timeseries  SampleTime=-1
  Log_TP_v2a_dcneg : ToWorkspace  VariableName=tp_v2a_dcneg  SaveFormat=Timeseries  SampleTime=-1
  Log_TP_v2b_dcneg : ToWorkspace  VariableName=tp_v2b_dcneg  SaveFormat=Timeseries  SampleTime=-1
  Log_TP_v2c_dcneg : ToWorkspace  VariableName=tp_v2c_dcneg  SaveFormat=Timeseries  SampleTime=-1
  Log_TP_vneutral_dcneg : ToWorkspace  VariableName=tp_vneutral_dcneg  SaveFormat=Timeseries  SampleTime=-1
  Log_UAB : ToWorkspace  VariableName=acac_uab  SaveFormat=Timeseries  SampleTime=-1
  Log_UBC : ToWorkspace  VariableName=acac_ubc  SaveFormat=Timeseries  SampleTime=-1
  Log_UCA : ToWorkspace  VariableName=acac_uca  SaveFormat=Timeseries  SampleTime=-1
  Log_VA : ToWorkspace  VariableName=acac_va  SaveFormat=Timeseries  SampleTime=-1
  Log_VB : ToWorkspace  VariableName=acac_vb  SaveFormat=Timeseries  SampleTime=-1
  Log_VC : ToWorkspace  VariableName=acac_vc  SaveFormat=Timeseries  SampleTime=-1
  Log_VDC : ToWorkspace  VariableName=acac_vdc  SaveFormat=Timeseries  SampleTime=-1
  Log_VIN : ToWorkspace  VariableName=acac_vin  SaveFormat=Timeseries  SampleTime=-1
  Return_Power_W : Product  Inputs=**
  wires:
  vin/1 -> Log_VIN/1
  iin/1 -> Log_IIN/1
  vdc/1 -> Log_VDC/1, Log_TP_conv2_dc_voltage/1, Return_Power_W/1
  pfc_duty/1 -> Log_PFC_DUTY/1
  inverter_modulation/1 -> Log_INVERTER_MODULATION/1
  ia/1 -> Log_IA/1
  va/1 -> Log_VA/1
  uab/1 -> Log_UAB/1
  ib/1 -> Log_IB/1
  vb/1 -> Log_VB/1
  ubc/1 -> Log_UBC/1
  ic/1 -> Log_IC/1
  vc/1 -> Log_VC/1
  uca/1 -> Log_UCA/1
  qfh/1 -> Log_QFH/1
  qfl/1 -> Log_QFL/1
  qsh/1 -> Log_QSH/1
  qsl/1 -> Log_QSL/1
  qah/1 -> Log_QAH/1
  qal/1 -> Log_QAL/1
  qbh/1 -> Log_QBH/1
  qbl/1 -> Log_QBL/1
  qch/1 -> Log_QCH/1
  qcl/1 -> Log_QCL/1
  precharge_bypass/1 -> Log_PRECHARGE_BYPASS/1
  final_precharge_bypass/1 -> Log_FINAL_PRECHARGE_BYPASS/1
  filter_current_a/1 -> Log_TP_filter_current_a/1
  filter_current_b/1 -> Log_TP_filter_current_b/1
  filter_current_c/1 -> Log_TP_filter_current_c/1
  id_source/1 -> Log_TP_id_source/1
  modA/1 -> Log_TP_modA/1
  modB/1 -> Log_TP_modB/1
  modC/1 -> Log_TP_modC/1
  conv2_ia/1 -> Log_TP_conv2_ia/1
  conv2_ib/1 -> Log_TP_conv2_ib/1
  conv2_ic/1 -> Log_TP_conv2_ic/1
  conv2_dc_return_current/1 -> Log_TP_conv2_dc_return_current/1, Return_Power_W/2
  Return_Power_W/1 -> Log_TP_return_power/1
  c2_gate_ah/1 -> Log_TP_c2_gate_ah/1
  c2_gate_al/1 -> Log_TP_c2_gate_al/1
  c2_gate_bh/1 -> Log_TP_c2_gate_bh/1
  c2_gate_bl/1 -> Log_TP_c2_gate_bl/1
  c2_gate_ch/1 -> Log_TP_c2_gate_ch/1
  c2_gate_cl/1 -> Log_TP_c2_gate_cl/1
  c2_id/1 -> Log_TP_c2_id/1
  c2_iq/1 -> Log_TP_c2_iq/1
  c2_id_ref/1 -> Log_TP_c2_id_ref/1
  c2_mod_peak/1 -> Log_TP_c2_mod_peak/1
  c2_current_limited/1 -> Log_TP_c2_current_limited/1
  vneutral_dcneg/1 -> Log_TP_vneutral_dcneg/1
  v2a_dcneg/1 -> Log_TP_v2a_dcneg/1
  v2b_dcneg/1 -> Log_TP_v2b_dcneg/1
  v2c_dcneg/1 -> Log_TP_v2c_dcneg/1
  v1a_dcneg/1 -> Log_TP_v1a_dcneg/1
  v1b_dcneg/1 -> Log_TP_v1b_dcneg/1
  v1c_dcneg/1 -> Log_TP_v1c_dcneg/1
  lconn_va/1 -> Log_TP_lconn_va/1
  lconn_vb/1 -> Log_TP_lconn_vb/1
  lconn_vc/1 -> Log_TP_lconn_vc/1

== matlab function energy_recovery_testbench_r2024a/Converter2_Control/Converter2_dq_Current_Control ==
  settings: updateMethod=DISCRETE  sampleTime=1e-6
  data: t input; gates output; va input; vb input; vc input; ia input; ib input; ic input; vdc input; iref_rms input; regen_enable input; id_meas output; iq_meas output; id_ref_used output; mod_peak output; current_limited output; Fout_Hz parameter
function [gates, id_meas, iq_meas, id_ref_used, mod_peak, current_limited] = converter2_controller(t, va, vb, vc, ia, ib, ic, vdc, iref_rms, regen_enable, Fout_Hz)
%#codegen
% Current ia,b,c is positive from Converter 1 through Lconn into Converter 2.
% Park d axis uses sin(theta); positive id thus absorbs real AC power.
% L di/dt = v1 - v2 - R i. All output gates have 1 us turn-on dead time.

persistent intD intQ idFilt iqFilt vdFilt vqFilt lastRaw onAge
if isempty(intD)
    intD=0.0; intQ=0.0;
    idFilt=0.0; iqFilt=0.0; vdFilt=0.0; vqFilt=0.0;
    lastRaw=false(1,6); onAge=zeros(1,6);
end
Ts=1e-6;
deadTime=1e-6;
fsw=12.6e3;
Lconn=0.003;
Rconn=0.05;
omega=2*pi*Fout_Hz;
wc=2*pi*300.0;
Kp=Lconn*wc;
Ki=Rconn*wc;
alpha=Ts/(1/(2*pi*1500)+Ts);
theta=omega*t;
sa=sin(theta); sb=sin(theta-2*pi/3); sc=sin(theta+2*pi/3);
ca=cos(theta); cb=cos(theta-2*pi/3); cc=cos(theta+2*pi/3);
idInstant=(2/3)*(ia*sa+ib*sb+ic*sc);
iqInstant=(2/3)*(ia*ca+ib*cb+ic*cc);
vdInstant=(2/3)*(va*sa+vb*sb+vc*sc);
vqInstant=(2/3)*(va*ca+vb*cb+vc*cc);
idFilt=idFilt+alpha*(idInstant-idFilt);
iqFilt=iqFilt+alpha*(iqInstant-iqFilt);
vdFilt=vdFilt+alpha*(vdInstant-vdFilt);
vqFilt=vqFilt+alpha*(vqInstant-vqFilt);
id_meas=idFilt;
iq_meas=iqFilt;

% Engineering protection: 2.2 A RMS is 10% above the 2 A rating.
current_limited=(iref_rms>2.2);
safeRefRms=min(max(iref_rms,0.0),2.2);
enabled=(regen_enable>0.5)&&(t>=0.25)&&(vdc>=50.0)&&(vdc<=70.0);
ramp=min(max((t-0.25)/0.15,0.0),1.0);
id_ref_used=sqrt(2.0)*safeRefRms*ramp;
if ~enabled
    id_ref_used=0.0;
end
ed=id_ref_used-idFilt;
eq=-iqFilt;

% For the stated Park basis: L*did/dt=vd1-vd2-R*id+L*w*iq;
%                         L*diq/dt=vq1-vq2-R*iq-L*w*id.
v2d=vdFilt+Lconn*omega*iqFilt-Kp*ed-intD;
v2q=vqFilt-Lconn*omega*idFilt-Kp*eq-intQ;
vLimit=0.95*max(vdc,1.0)/2.0;
vNorm=hypot(v2d,v2q);
if vNorm>vLimit
    scale=vLimit/vNorm;
    v2d=v2d*scale; v2q=v2q*scale;
else
    intD=min(max(intD+Ki*Ts*ed,-8.0),8.0);
    intQ=min(max(intQ+Ki*Ts*eq,-8.0),8.0);
end

v2a=v2d*sa+v2q*ca;
v2b=v2d*sb+v2q*cb;
v2c=v2d*sc+v2q*cc;
ma=min(max(2*v2a/max(vdc,1.0),-0.95),0.95);
mb=min(max(2*v2b/max(vdc,1.0),-0.95),0.95);
mc=min(max(2*v2c/max(vdc,1.0),-0.95),0.95);
mod_peak=max(max(abs(ma),abs(mb)),abs(mc));

phase=mod(t*fsw,1.0);
carrier=1.0-4.0*abs(phase-0.5);
raw=false(1,6);
if enabled
    ah=ma>carrier; bh=mb>carrier; ch=mc>carrier;
    raw(1)=ah; raw(2)=~ah;
    raw(3)=bh; raw(4)=~bh;
    raw(5)=ch; raw(6)=~ch;
end
gates=false(6,1);
for k=1:6
    if raw(k)
        if lastRaw(k)
            onAge(k)=min(onAge(k)+Ts,deadTime);
        else
            onAge(k)=0.0;
        end
        gates(k)=onAge(k)>=deadTime;
    else
        onAge(k)=0.0;
        gates(k)=false;
    end
    lastRaw(k)=raw(k);
end
end
